simulink model "New_entropy"  (Simulink 7.9)
settings: Solver=FixedStepDiscrete  StartTime=0.0  StopTime=10  FixedStep=1  RelTol=1e-3
undefined symbols (not defined in the file): Carnot_entropy_Callbacks
settings Model: Creator=awohlfei  LastModifiedBy=awohlfei

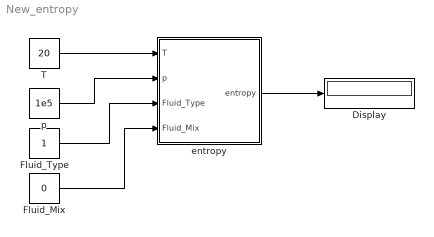
== system New_entropy ==
  Display : Display
  Fluid_Mix : Constant  Value=0
  Fluid_Type : Constant
  T : Constant  Value=20
  entropy : Subsystem  LoadFcn=Carnot_entropy_Callbacks('LoadFcn');  InitFcn=load('THB.mat');  VariantObject=CarlibClassic  mask(entropy){INPUTARGUMENTS=state variables (classic), DEBUGLEVEL=WARNING, MAXTOTALMESSAGES=inf, MAXCONSECUTIVEMESSAGES=inf, WRITETOFILE=0, FILENAME='errors.txt'}
      mask prompts: INPUTARGUMENTS "Input arguments"; DEBUGLEVEL "Debug level"; MAXTOTALMESSAGES "maximum number of total warning"; MAXCONSECUTIVEMESSAGES "maximum number of consecutive warnings"; WRITETOFILE "write messages to file"; FILENAME "filename for error messages"
      mask help:
      | The block calculates the entropy  [J/kgK] of the fluid.
      | The block calls the function "entropy" in the
      | CARNOT library "carlib".
      | Definition of the fluid types
      | fluid-ID  material           remarks on fluid mix
      | 1           water              vapourcontent in the 2-phase region
      | 2           air                   is (kg water) / (kg air)
      | 3           cotton oil
      | 4           silicone oil
      | 5           water-glycol    gives the volume partition [0..1] of glycol
      | 6           tyfocor_LS      only available in liquid phase
      mask init:
      | %Inports
      | Carnot_entropy_Callbacks('CreateInports');
      | 
      | %global debug level
      | [DEBUGLEVEL, MAXTOTALMESSAGES, MAXCONSECUTIVEMESSAGES, WRITETOFILE, FILENAME] = Carnot_entropy_Callbacks('CheckDebugLevels', DEBUGLEVEL, MAXTOTALMESSAGES, MAXCONSECUTIVEMESSAGES, WRITETOFILE, FILENAME);
      mask Help: eval('man(''entropy'')')
      mask StyleString: popup(state variables (classic)|THB|THV),popup(DEBUG|INFO|WARNING|ERROR|FATAL|NONE),edit,edit,edit,edit
      mask CallbackString: Carnot_entropy_Callbacks('MaskVisibilities');|||||
      mask TabNameString: Parameters,Debugging,Debugging,Debugging,Debugging,Debugging
  p : Constant  Value=1e5
  wires:
  T/1 -> entropy/1(T)
  p/1 -> entropy/2(p)
  Fluid_Type/1 -> entropy/3(Fluid_Type)
  Fluid_Mix/1 -> entropy/4(Fluid_Mix)
  entropy/1(entropy) -> Display/1

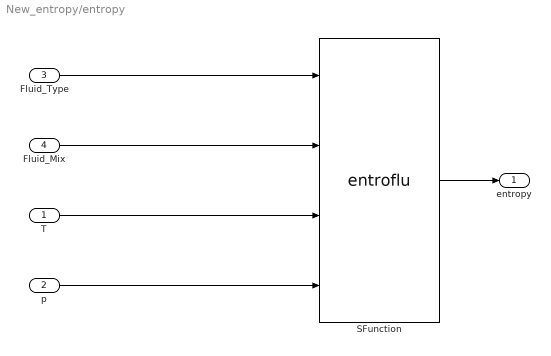
== system New_entropy/entropy ==
  T : Inport
  p : Inport  Port=2
  Fluid_Type : Inport  Port=3
  Fluid_Mix : Inport  Port=4
  SFunction : S-Function  FunctionName=entroflu  Parameters=DEBUGLEVEL,MAXTOTALMESSAGES,MAXCONSECUTIVEMESSAGES,WRITETOFILE,FILENAME  EnableBusSupport=off
  entropy : Outport
  wires:
  SFunction/1 -> entropy/1
  T/1 -> SFunction/3
  p/1 -> SFunction/4
  Fluid_Type/1 -> SFunction/1
  Fluid_Mix/1 -> SFunction/2
